simulink model "sysout"  (R2019a)
settings: Solver=VariableStepAuto  StartTime=0.0  StopTime=10.0  FixedStep=1e-3  MaxStep=1e-2  RelTol=1e-4  AbsTol=1e-4
values from neighbouring files (symbols this model uses):
  den = SYS.Denominator    [sys_ident.m]
  den1 = [8 115 13]    [sys_ident.m]
  num = SYS.Numerator    [sys_ident.m]
  num1 = [11.25]    [sys_ident.m]
settings Model: Creator=DELL  LastModifiedBy=DELL

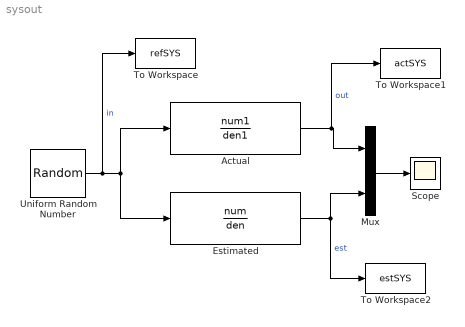
== system sysout ==
  Actual : TransferFcn  Numerator=num1  Denominator=den1
  Estimated : TransferFcn  Numerator=num  Denominator=den
  Mux : Mux  Inputs=2
  Scope : Scope
  To Workspace : ToWorkspace  VariableName=refSYS  SampleTime=-1
  To Workspace1 : ToWorkspace  VariableName=actSYS  SampleTime=-1
  To Workspace2 : ToWorkspace  VariableName=estSYS  SampleTime=-1
  Uniform Random Number : UniformRandomNumber  SampleTime=1e-3
  wires:
  Uniform Random Number/1 -> To Workspace/1, Actual/1, Estimated/1  "in"
  Mux/1 -> Scope/1
  Actual/1 -> To Workspace1/1, Mux/1  "out"
  Estimated/1 -> To Workspace2/1, Mux/2  "est"
